simulink model "test_2020a"  (R2020a)
settings: Solver=FixedStepAuto  StartTime=0.0  StopTime=10.0  RelTol=1e-3
model workspace (MAT data in the model file):
  SL_ROS_VariableLengthArrays_MaxSizes.CommonInfo.ArrayTruncateAction = 'EmitWarning'
  SL_ROS_VariableLengthArrays_MaxSizes.MsgTypeMap = containers.Map
  SL_ROS_VariableLengthArrays_MaxSizes.MsgTypeMap.serialization.keys = {'sensor_msgs/Image'}
  SL_ROS_VariableLengthArrays_MaxSizes.MsgTypeMap.serialization.values{1}(1).PropertyName = 'Data'
  SL_ROS_VariableLengthArrays_MaxSizes.MsgTypeMap.serialization.values{1}(1).DataType = 'uint8'
  SL_ROS_VariableLengthArrays_MaxSizes.MsgTypeMap.serialization.values{1}(1).MaxLength = 3121200
  SL_ROS_VariableLengthArrays_MaxSizes.MsgTypeMap.serialization.values{1}(2).PropertyName = 'Encoding'
  SL_ROS_VariableLengthArrays_MaxSizes.MsgTypeMap.serialization.values{1}(2).DataType = 'uint8'
  SL_ROS_VariableLengthArrays_MaxSizes.MsgTypeMap.serialization.values{1}(2).MaxLength = 128
  SL_ROS_VariableLengthArrays_MaxSizes.MsgTypeMap.serialization.uniformity = 0
  SL_ROS_VariableLengthArrays_MaxSizes.MsgTypeMap.serialization.keyType = 'char'
  SL_ROS_VariableLengthArrays_MaxSizes.MsgTypeMap.serialization.valueType = 'any'
undefined symbols (not defined in the file): gray
libraries: robotlib x2
settings Model: Creator=shiva  LastModifiedBy=Ali

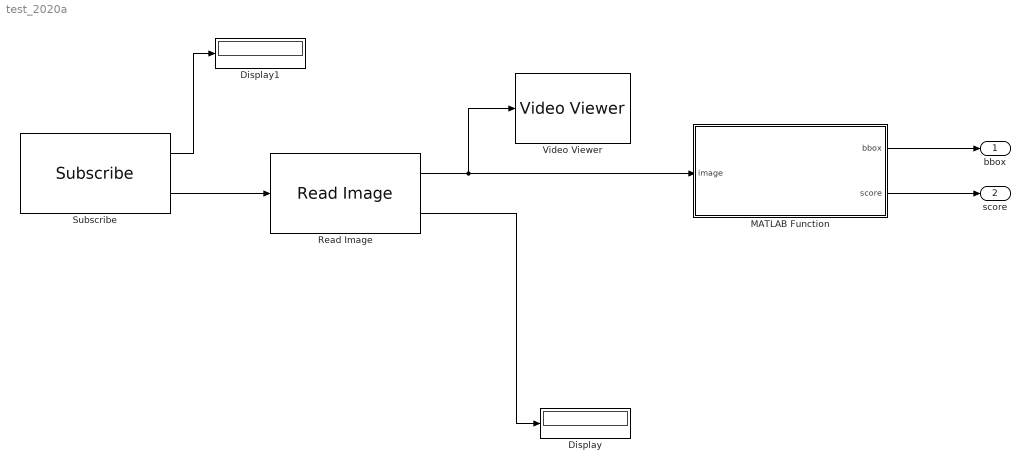
== system test_2020a ==
  Display : Display
  Display1 : Display
  MATLAB Function : MATLAB Function  TreatAsAtomicUnit=on
  Read Image : robotlib/Read Image  MaximumImageSize=[1020, 1020]  ImageEncoding=rgb8  ShowAlphaOutput=off  ShowErrorCodeOutput=on  VariableSizeOutputs=off
      settings: SourceProductBaseCode=RR
  Subscribe : robotlib/Subscribe  topicSource=Select from ROS network  topic=/robot_sensor/camera/image_raw  messageType=sensor_msgs/Image  SampleTime=-1  legacyBusStruct=off  messageQueueLength=1
  Video Viewer : VideoViewer  colormapValue=gray(256)  FigPos=[253 634.8 418.4 304]
  bbox : Outport
  score : Outport  Port=2
  wires:
  Subscribe/2 -> Read Image/1
  Read Image/2 -> Display/1
  Read Image/1 -> MATLAB Function/1(image), Video Viewer/1
  Subscribe/1 -> Display1/1
  MATLAB Function/2(score) -> score/1
  MATLAB Function/1(bbox) -> bbox/1

== matlab function test_2020a/MATLAB Function ==
  data: image input; bbox output; score output
function [bbox, score] = yolov2_detect(image)
bbox = zeros(1, 4);
score = 0;

imageResized = imresize(image,[224, 224]);

persistent yolov2Obj;

if isempty(yolov2Obj)
    yolov2Obj = coder.loadDeepLearningNetwork('yoloResNet50_det.mat');
end

[bboxes, scores] = yolov2Obj.detect(imageResized,'Threshold',0.5);


if ~isempty(bboxes)
    bbox = bboxes(1, :);
    score = double(scores(1));
end
end
